simulink model "Kubon_lab6_sim"  (R2020b)
settings: Solver=VariableStepAuto  StartTime=0.0  StopTime=20.0  RelTol=1e-3
values from neighbouring files (symbols this model uses):
  A1 = [0,-6/7,-16/7,47/7]    [Kubon_lab4.m]    (also in Kubon_lab6.m = 1; Kubon_lab6_test.m = 1; Kubon_lab7.m = 4; Kubon_lab8.m = 4)
  a1 = 1    [Kubon_lab4.m]    (also in Kubon_lab6.m = Aw1*sqrt(2*g/H1); Kubon_lab6_test.m = Aw1*sqrt(2*g/H1); Kubon_lab7.m = Aw1*sqrt(2*g/(H1-H2)); Kubon_lab8.m = Aw1*sqrt(2*g/(H1-H2)))
  A2 = 7    [Kubon_lab6.m]    (also in Kubon_lab6_test.m; Kubon_lab7.m = 4; Kubon_lab8.m = 4)
  a2 = Aw2*sqrt(2*g/H2)    [Kubon_lab6.m]    (also in Kubon_lab6_test.m; Kubon_lab7.m; Kubon_lab8.m)
  d1 = 0.1*fwe1max    [Kubon_lab6.m]    (also in Kubon_lab7.m = 0; Kubon_lab8.m = 0)
  fwe1 = fwe1w(i)    [Kubon_lab6.m]    (also in Kubon_lab6_test.m; Kubon_lab7.m = 0.1*fwe1max; Kubon_lab8.m = 0.1*fwe1max)
  fwe2 = fwe2w(i)    [Kubon_lab6.m]    (also in Kubon_lab6_test.m; Kubon_lab7.m; Kubon_lab8.m)
  h10 = fwe1/a1    [Kubon_lab6.m]    (also in Kubon_lab6_test.m; Kubon_lab7.m = (1/(2*g))*(fwe1/Aw1)^2 + (1/(2*g))*(((fwe2+fwe1)/Aw2)^2); Kubon_lab8.m = fwe1/a1+(fwe2+fwe1)/a2)
  h20 = (fwe1+fwe2)/a2    [Kubon_lab6.m]    (also in Kubon_lab6_test.m; Kubon_lab7.m = 1/(2*g)*(((fwe1+fwe2)/Aw2)^2); Kubon_lab8.m = (fwe2+fwe1)/a2)
  t0 = 50.0    (= 50)    [Kubon_lab10.m]    (also in Kubon_lab4.m = 5; Kubon_lab5.m = 0; Kubon_lab6.m = 5; Kubon_lab6_test.m = 0)
settings Model: Creator=pkubo  LastModifiedBy=pkubo

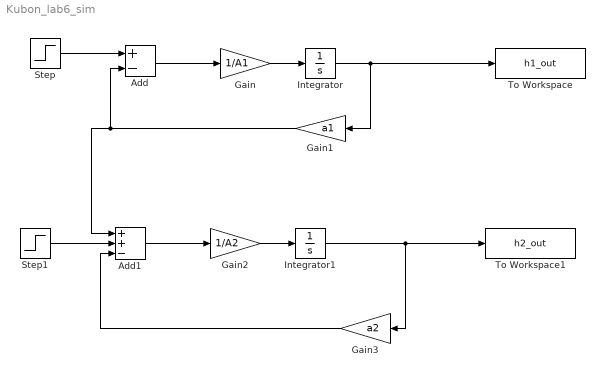
== system Kubon_lab6_sim ==
  Add : Sum  Inputs=+-
  Add1 : Sum  Inputs=++-
  Gain : Gain  Gain=1/A1
  Gain1 : Gain  Gain=a1
  Gain2 : Gain  Gain=1/A2
  Gain3 : Gain  Gain=a2
  Integrator : Integrator  InitialCondition=h10
  Integrator1 : Integrator  InitialCondition=h20
  Step : Step  Time=t0  Before=fwe1  After=fwe1+ d1  SampleTime=0
  Step1 : Step  Time=t0  Before=fwe2  After=fwe2+ d1  SampleTime=0
  To Workspace : ToWorkspace  VariableName=h1_out  SampleTime=-1
  To Workspace1 : ToWorkspace  VariableName=h2_out  SampleTime=-1
  wires:
  Step/1 -> Add/1
  Add/1 -> Gain/1
  Gain/1 -> Integrator/1
  Integrator/1 -> To Workspace/1, Gain1/1
  Add1/1 -> Gain2/1
  Gain2/1 -> Integrator1/1
  Integrator1/1 -> To Workspace1/1, Gain3/1
  Gain1/1 -> Add1/1, Add/2
  Step1/1 -> Add1/2
  Gain3/1 -> Add1/3
